simulink model "14_bus"  (R2024a)
settings: Solver=VariableStepAuto  StartTime=0.0  StopTime=1  RelTol=1e-3
undefined symbols (not defined in the file): D1, Delta
libraries: spsRMSLib x186, simulink_extras x171, spsThreePhaseVIMeasurementLib x94, spsThreePhaseBreakerLib x62, spsThreePhaseSeriesRLCBranchLib x20, spsThreePhaseSeriesRLCLoadLib x12, spsThreePhaseSourceLib x5, spsLoadFlowBusLib x5, spsStairGeneratorLib x5, spsThreePhaseTransformerTwoWindingsLib x5, spsThreePhaseFaultLib x5, sps_lib x1
(part 3 of 6)

== system 14_bus/Subsystem35 ==
  Subsystem1 : Subsystem
  Three-Phase Breaker26 : spsThreePhaseBreakerLib/Three-Phase Breaker  InitialState=closed  SwitchA=on  SwitchB=on  SwitchC=on  SwitchTimes="[1/60  5/60]"  External=on  BreakerResistance=0.01  SnubberResistance=1e6  SnubberCapacitance=inf  Measurements=None
  VI13 : spsThreePhaseVIMeasurementLib/Three-Phase V-I Measurement  VoltageMeasurement=no  SetLabelV=off  LabelV=Vabc  Vpu=off  VpuLL=off  CurrentMeasurement=yes  SetLabelI=on  LabelI=I109  Ipu=off  Pbase=100e6  Vbase=500e3  OutputType=Complex  PhasorSimulation=off  PSBequivalent=0
  A : PMIOPort  Side=Left
  B : PMIOPort  Port=2  Side=Left
  C : PMIOPort  Port=3  Side=Left
  a : PMIOPort  Port=4  Side=Right
  b : PMIOPort  Port=5  Side=Right
  c : PMIOPort  Port=6  Side=Right
  wires:
  Subsystem1/1(Out1) -> Three-Phase Breaker26/1
  [I109] -> Subsystem1/1(Iabc1)
  connections:
  VI13/LConn1 -- A/RConn1
  Three-Phase Breaker26/LConn2 -- VI13/RConn2
  Three-Phase Breaker26/LConn3 -- VI13/RConn3
  Three-Phase Breaker26/LConn1 -- VI13/RConn1
  VI13/LConn2 -- B/RConn1
  Three-Phase Breaker26/RConn1 -- a/RConn1
  VI13/LConn3 -- C/RConn1
  Three-Phase Breaker26/RConn2 -- b/RConn1
  Three-Phase Breaker26/RConn3 -- c/RConn1

== system 14_bus/Subsystem36 ==
  Subsystem1 : Subsystem
  Three-Phase Breaker26 : spsThreePhaseBreakerLib/Three-Phase Breaker  InitialState=closed  SwitchA=on  SwitchB=on  SwitchC=on  SwitchTimes="[1/60  5/60]"  External=on  BreakerResistance=0.01  SnubberResistance=1e6  SnubberCapacitance=inf  Measurements=None
  VI13 : spsThreePhaseVIMeasurementLib/Three-Phase V-I Measurement  VoltageMeasurement=no  SetLabelV=off  LabelV=Vabc  Vpu=off  VpuLL=off  CurrentMeasurement=yes  SetLabelI=on  LabelI=I910  Ipu=off  Pbase=100e6  Vbase=500e3  OutputType=Complex  PhasorSimulation=off  PSBequivalent=0
  A : PMIOPort  Side=Left
  B : PMIOPort  Port=2  Side=Left
  C : PMIOPort  Port=3  Side=Left
  a : PMIOPort  Port=4  Side=Right
  b : PMIOPort  Port=5  Side=Right
  c : PMIOPort  Port=6  Side=Right
  wires:
  Subsystem1/1(Out1) -> Three-Phase Breaker26/1
  [I910] -> Subsystem1/1(Iabc1)
  connections:
  VI13/LConn1 -- A/RConn1
  Three-Phase Breaker26/LConn2 -- VI13/RConn2
  Three-Phase Breaker26/LConn3 -- VI13/RConn3
  Three-Phase Breaker26/LConn1 -- VI13/RConn1
  VI13/LConn2 -- B/RConn1
  Three-Phase Breaker26/RConn1 -- a/RConn1
  VI13/LConn3 -- C/RConn1
  Three-Phase Breaker26/RConn2 -- b/RConn1
  Three-Phase Breaker26/RConn3 -- c/RConn1

== system 14_bus/Subsystem37 ==
  Subsystem1 : Subsystem
  Three-Phase Breaker26 : spsThreePhaseBreakerLib/Three-Phase Breaker  InitialState=closed  SwitchA=on  SwitchB=on  SwitchC=on  SwitchTimes="[1/60  5/60]"  External=on  BreakerResistance=0.01  SnubberResistance=1e6  SnubberCapacitance=inf  Measurements=None
  VI13 : spsThreePhaseVIMeasurementLib/Three-Phase V-I Measurement  VoltageMeasurement=no  SetLabelV=off  LabelV=Vabc  Vpu=off  VpuLL=off  CurrentMeasurement=yes  SetLabelI=on  LabelI=I1110  Ipu=off  Pbase=100e6  Vbase=500e3  OutputType=Complex  PhasorSimulation=off  PSBequivalent=0
  A : PMIOPort  Side=Left
  B : PMIOPort  Port=2  Side=Left
  C : PMIOPort  Port=3  Side=Left
  a : PMIOPort  Port=4  Side=Right
  b : PMIOPort  Port=5  Side=Right
  c : PMIOPort  Port=6  Side=Right
  wires:
  Subsystem1/1(Out1) -> Three-Phase Breaker26/1
  [I1110] -> Subsystem1/1(Iabc1)
  connections:
  VI13/LConn1 -- A/RConn1
  Three-Phase Breaker26/LConn2 -- VI13/RConn2
  Three-Phase Breaker26/LConn3 -- VI13/RConn3
  Three-Phase Breaker26/LConn1 -- VI13/RConn1
  VI13/LConn2 -- B/RConn1
  Three-Phase Breaker26/RConn1 -- a/RConn1
  VI13/LConn3 -- C/RConn1
  Three-Phase Breaker26/RConn2 -- b/RConn1
  Three-Phase Breaker26/RConn3 -- c/RConn1

== system 14_bus/Subsystem38 ==
  Subsystem1 : Subsystem
  Three-Phase Breaker26 : spsThreePhaseBreakerLib/Three-Phase Breaker  InitialState=closed  SwitchA=on  SwitchB=on  SwitchC=on  SwitchTimes="[1/60  5/60]"  External=on  BreakerResistance=0.01  SnubberResistance=1e6  SnubberCapacitance=inf  Measurements=None
  VI13 : spsThreePhaseVIMeasurementLib/Three-Phase V-I Measurement  VoltageMeasurement=no  SetLabelV=off  LabelV=Vabc  Vpu=off  VpuLL=off  CurrentMeasurement=yes  SetLabelI=on  LabelI=I1011  Ipu=off  Pbase=100e6  Vbase=500e3  OutputType=Complex  PhasorSimulation=off  PSBequivalent=0
  A : PMIOPort  Side=Left
  B : PMIOPort  Port=2  Side=Left
  C : PMIOPort  Port=3  Side=Left
  a : PMIOPort  Port=4  Side=Right
  b : PMIOPort  Port=5  Side=Right
  c : PMIOPort  Port=6  Side=Right
  wires:
  Subsystem1/1(Out1) -> Three-Phase Breaker26/1
  [I1011] -> Subsystem1/1(Iabc1)
  connections:
  VI13/LConn1 -- A/RConn1
  Three-Phase Breaker26/LConn2 -- VI13/RConn2
  Three-Phase Breaker26/LConn3 -- VI13/RConn3
  Three-Phase Breaker26/LConn1 -- VI13/RConn1
  VI13/LConn2 -- B/RConn1
  Three-Phase Breaker26/RConn1 -- a/RConn1
  VI13/LConn3 -- C/RConn1
  Three-Phase Breaker26/RConn2 -- b/RConn1
  Three-Phase Breaker26/RConn3 -- c/RConn1

== system 14_bus/Subsystem39 ==
  Subsystem1 : Subsystem
  Three-Phase Breaker26 : spsThreePhaseBreakerLib/Three-Phase Breaker  InitialState=closed  SwitchA=on  SwitchB=on  SwitchC=on  SwitchTimes="[1/60  5/60]"  External=on  BreakerResistance=0.01  SnubberResistance=1e6  SnubberCapacitance=inf  Measurements=None
  VI13 : spsThreePhaseVIMeasurementLib/Three-Phase V-I Measurement  VoltageMeasurement=no  SetLabelV=off  LabelV=Vabc  Vpu=off  VpuLL=off  CurrentMeasurement=yes  SetLabelI=on  LabelI=I116  Ipu=off  Pbase=100e6  Vbase=500e3  OutputType=Complex  PhasorSimulation=off  PSBequivalent=0
  A : PMIOPort  Side=Left
  B : PMIOPort  Port=2  Side=Left
  C : PMIOPort  Port=3  Side=Left
  a : PMIOPort  Port=4  Side=Right
  b : PMIOPort  Port=5  Side=Right
  c : PMIOPort  Port=6  Side=Right
  wires:
  Subsystem1/1(Out1) -> Three-Phase Breaker26/1
  [I116] -> Subsystem1/1(Iabc1)
  connections:
  VI13/LConn1 -- A/RConn1
  Three-Phase Breaker26/LConn2 -- VI13/RConn2
  Three-Phase Breaker26/LConn3 -- VI13/RConn3
  Three-Phase Breaker26/LConn1 -- VI13/RConn1
  VI13/LConn2 -- B/RConn1
  Three-Phase Breaker26/RConn1 -- a/RConn1
  VI13/LConn3 -- C/RConn1
  Three-Phase Breaker26/RConn2 -- b/RConn1
  Three-Phase Breaker26/RConn3 -- c/RConn1

== system 14_bus/Subsystem4 ==
  Subsystem25 : Subsystem
  Three-Phase Breaker26 : spsThreePhaseBreakerLib/Three-Phase Breaker  InitialState=closed  SwitchA=on  SwitchB=on  SwitchC=on  SwitchTimes="[1/60  5/60]"  External=on  BreakerResistance=0.01  SnubberResistance=1e6  SnubberCapacitance=inf  Measurements=None
  VI13 : spsThreePhaseVIMeasurementLib/Three-Phase V-I Measurement  VoltageMeasurement=no  SetLabelV=off  LabelV=Vabc  Vpu=off  VpuLL=off  CurrentMeasurement=yes  SetLabelI=on  LabelI=I74  Ipu=off  Pbase=100e6  Vbase=500e3  OutputType=Complex  PhasorSimulation=off  PSBequivalent=0
  A : PMIOPort  Side=Left
  B : PMIOPort  Port=2  Side=Left
  C : PMIOPort  Port=3  Side=Left
  a : PMIOPort  Port=4  Side=Right
  b : PMIOPort  Port=5  Side=Right
  c : PMIOPort  Port=6  Side=Right
  wires:
  Subsystem25/1(Out1) -> Three-Phase Breaker26/1
  [I74] -> Subsystem25/1(Iabc1)
  connections:
  VI13/LConn3 -- C/RConn1
  Three-Phase Breaker26/LConn3 -- VI13/RConn3
  Three-Phase Breaker26/RConn2 -- b/RConn1
  VI13/LConn1 -- A/RConn1
  Three-Phase Breaker26/RConn1 -- a/RConn1
  Three-Phase Breaker26/LConn1 -- VI13/RConn1
  Three-Phase Breaker26/LConn2 -- VI13/RConn2
  Three-Phase Breaker26/RConn3 -- c/RConn1
  VI13/LConn2 -- B/RConn1

== system 14_bus/Subsystem40 ==
  Subsystem1 : Subsystem
  Three-Phase Breaker26 : spsThreePhaseBreakerLib/Three-Phase Breaker  InitialState=closed  SwitchA=on  SwitchB=on  SwitchC=on  SwitchTimes="[1/60  5/60]"  External=on  BreakerResistance=0.01  SnubberResistance=1e6  SnubberCapacitance=inf  Measurements=None
  VI13 : spsThreePhaseVIMeasurementLib/Three-Phase V-I Measurement  VoltageMeasurement=no  SetLabelV=off  LabelV=Vabc  Vpu=off  VpuLL=off  CurrentMeasurement=yes  SetLabelI=on  LabelI=I611  Ipu=off  Pbase=100e6  Vbase=500e3  OutputType=Complex  PhasorSimulation=off  PSBequivalent=0
  A : PMIOPort  Side=Left
  B : PMIOPort  Port=2  Side=Left
  C : PMIOPort  Port=3  Side=Left
  a : PMIOPort  Port=4  Side=Right
  b : PMIOPort  Port=5  Side=Right
  c : PMIOPort  Port=6  Side=Right
  wires:
  Subsystem1/1(Out1) -> Three-Phase Breaker26/1
  [I611] -> Subsystem1/1(Iabc1)
  connections:
  VI13/LConn1 -- A/RConn1
  Three-Phase Breaker26/LConn2 -- VI13/RConn2
  Three-Phase Breaker26/LConn3 -- VI13/RConn3
  Three-Phase Breaker26/LConn1 -- VI13/RConn1
  VI13/LConn2 -- B/RConn1
  Three-Phase Breaker26/RConn1 -- a/RConn1
  VI13/LConn3 -- C/RConn1
  Three-Phase Breaker26/RConn2 -- b/RConn1
  Three-Phase Breaker26/RConn3 -- c/RConn1

== system 14_bus/Subsystem41 ==
  Subsystem1 : Subsystem
  Three-Phase Breaker26 : spsThreePhaseBreakerLib/Three-Phase Breaker  InitialState=closed  SwitchA=on  SwitchB=on  SwitchC=on  SwitchTimes="[1/60  5/60]"  External=on  BreakerResistance=0.01  SnubberResistance=1e6  SnubberCapacitance=inf  Measurements=None
  VI13 : spsThreePhaseVIMeasurementLib/Three-Phase V-I Measurement  VoltageMeasurement=no  SetLabelV=off  LabelV=Vabc  Vpu=off  VpuLL=off  CurrentMeasurement=yes  SetLabelI=on  LabelI=IL6  Ipu=off  Pbase=100e6  Vbase=500e3  OutputType=Complex  PhasorSimulation=off  PSBequivalent=0
  A : PMIOPort  Side=Left
  B : PMIOPort  Port=2  Side=Left
  C : PMIOPort  Port=3  Side=Left
  a : PMIOPort  Port=4  Side=Right
  b : PMIOPort  Port=5  Side=Right
  c : PMIOPort  Port=6  Side=Right
  wires:
  Subsystem1/1(Out1) -> Three-Phase Breaker26/1
  [IL6] -> Subsystem1/1(Iabc1)
  connections:
  VI13/LConn1 -- A/RConn1
  Three-Phase Breaker26/LConn2 -- VI13/RConn2
  Three-Phase Breaker26/LConn3 -- VI13/RConn3
  Three-Phase Breaker26/LConn1 -- VI13/RConn1
  VI13/LConn2 -- B/RConn1
  Three-Phase Breaker26/RConn1 -- a/RConn1
  VI13/LConn3 -- C/RConn1
  Three-Phase Breaker26/RConn2 -- b/RConn1
  Three-Phase Breaker26/RConn3 -- c/RConn1

== system 14_bus/Subsystem42 ==
  Subsystem1 : Subsystem
  Three-Phase Breaker26 : spsThreePhaseBreakerLib/Three-Phase Breaker  InitialState=closed  SwitchA=on  SwitchB=on  SwitchC=on  SwitchTimes="[1/60  5/60]"  External=on  BreakerResistance=0.01  SnubberResistance=1e6  SnubberCapacitance=inf  Measurements=None
  VI13 : spsThreePhaseVIMeasurementLib/Three-Phase V-I Measurement  VoltageMeasurement=no  SetLabelV=off  LabelV=Vabc  Vpu=off  VpuLL=off  CurrentMeasurement=yes  SetLabelI=on  LabelI=I56  Ipu=off  Pbase=100e6  Vbase=500e3  OutputType=Complex  PhasorSimulation=off  PSBequivalent=0
  A : PMIOPort  Side=Left
  B : PMIOPort  Port=2  Side=Left
  C : PMIOPort  Port=3  Side=Left
  a : PMIOPort  Port=4  Side=Right
  b : PMIOPort  Port=5  Side=Right
  c : PMIOPort  Port=6  Side=Right
  wires:
  Subsystem1/1(Out1) -> Three-Phase Breaker26/1
  [I56] -> Subsystem1/1(Iabc1)
  connections:
  VI13/LConn1 -- A/RConn1
  Three-Phase Breaker26/LConn2 -- VI13/RConn2
  Three-Phase Breaker26/LConn3 -- VI13/RConn3
  Three-Phase Breaker26/LConn1 -- VI13/RConn1
  VI13/LConn2 -- B/RConn1
  Three-Phase Breaker26/RConn1 -- a/RConn1
  VI13/LConn3 -- C/RConn1
  Three-Phase Breaker26/RConn2 -- b/RConn1
  Three-Phase Breaker26/RConn3 -- c/RConn1

== system 14_bus/Subsystem43 ==
  Subsystem1 : Subsystem
  Three-Phase Breaker26 : spsThreePhaseBreakerLib/Three-Phase Breaker  InitialState=closed  SwitchA=on  SwitchB=on  SwitchC=on  SwitchTimes="[1/60  5/60]"  External=on  BreakerResistance=0.01  SnubberResistance=1e6  SnubberCapacitance=inf  Measurements=None
  VI13 : spsThreePhaseVIMeasurementLib/Three-Phase V-I Measurement  VoltageMeasurement=no  SetLabelV=off  LabelV=Vabc  Vpu=off  VpuLL=off  CurrentMeasurement=yes  SetLabelI=on  LabelI=I65  Ipu=off  Pbase=100e6  Vbase=500e3  OutputType=Complex  PhasorSimulation=off  PSBequivalent=0
  A : PMIOPort  Side=Left
  B : PMIOPort  Port=2  Side=Left
  C : PMIOPort  Port=3  Side=Left
  a : PMIOPort  Port=4  Side=Right
  b : PMIOPort  Port=5  Side=Right
  c : PMIOPort  Port=6  Side=Right
  wires:
  Subsystem1/1(Out1) -> Three-Phase Breaker26/1
  [I65] -> Subsystem1/1(Iabc1)
  connections:
  VI13/LConn1 -- A/RConn1
  Three-Phase Breaker26/LConn2 -- VI13/RConn2
  Three-Phase Breaker26/LConn3 -- VI13/RConn3
  Three-Phase Breaker26/LConn1 -- VI13/RConn1
  VI13/LConn2 -- B/RConn1
  Three-Phase Breaker26/RConn1 -- a/RConn1
  VI13/LConn3 -- C/RConn1
  Three-Phase Breaker26/RConn2 -- b/RConn1
  Three-Phase Breaker26/RConn3 -- c/RConn1

== system 14_bus/Subsystem44 ==
  Subsystem1 : Subsystem
  Three-Phase Breaker26 : spsThreePhaseBreakerLib/Three-Phase Breaker  InitialState=closed  SwitchA=on  SwitchB=on  SwitchC=on  SwitchTimes="[1/60  5/60]"  External=on  BreakerResistance=0.01  SnubberResistance=1e6  SnubberCapacitance=inf  Measurements=None
  VI13 : spsThreePhaseVIMeasurementLib/Three-Phase V-I Measurement  VoltageMeasurement=no  SetLabelV=off  LabelV=Vabc  Vpu=off  VpuLL=off  CurrentMeasurement=yes  SetLabelI=on  LabelI=I149  Ipu=off  Pbase=100e6  Vbase=500e3  OutputType=Complex  PhasorSimulation=off  PSBequivalent=0
  A : PMIOPort  Side=Left
  B : PMIOPort  Port=2  Side=Left
  C : PMIOPort  Port=3  Side=Left
  a : PMIOPort  Port=4  Side=Right
  b : PMIOPort  Port=5  Side=Right
  c : PMIOPort  Port=6  Side=Right
  wires:
  Subsystem1/1(Out1) -> Three-Phase Breaker26/1
  [I149] -> Subsystem1/1(Iabc1)
  connections:
  VI13/LConn1 -- A/RConn1
  Three-Phase Breaker26/LConn2 -- VI13/RConn2
  Three-Phase Breaker26/LConn3 -- VI13/RConn3
  Three-Phase Breaker26/LConn1 -- VI13/RConn1
  VI13/LConn2 -- B/RConn1
  Three-Phase Breaker26/RConn1 -- a/RConn1
  VI13/LConn3 -- C/RConn1
  Three-Phase Breaker26/RConn2 -- b/RConn1
  Three-Phase Breaker26/RConn3 -- c/RConn1

== system 14_bus/Subsystem45 ==
  Subsystem1 : Subsystem
  Three-Phase Breaker26 : spsThreePhaseBreakerLib/Three-Phase Breaker  InitialState=closed  SwitchA=on  SwitchB=on  SwitchC=on  SwitchTimes="[1/60  5/60]"  External=on  BreakerResistance=0.01  SnubberResistance=1e6  SnubberCapacitance=inf  Measurements=None
  VI13 : spsThreePhaseVIMeasurementLib/Three-Phase V-I Measurement  VoltageMeasurement=no  SetLabelV=off  LabelV=Vabc  Vpu=off  VpuLL=off  CurrentMeasurement=yes  SetLabelI=on  LabelI=I914  Ipu=off  Pbase=100e6  Vbase=500e3  OutputType=Complex  PhasorSimulation=off  PSBequivalent=0
  A : PMIOPort  Side=Left
  B : PMIOPort  Port=2  Side=Left
  C : PMIOPort  Port=3  Side=Left
  a : PMIOPort  Port=4  Side=Right
  b : PMIOPort  Port=5  Side=Right
  c : PMIOPort  Port=6  Side=Right
  wires:
  Subsystem1/1(Out1) -> Three-Phase Breaker26/1
  [I914] -> Subsystem1/1(Iabc1)
  connections:
  VI13/LConn1 -- A/RConn1
  Three-Phase Breaker26/LConn2 -- VI13/RConn2
  Three-Phase Breaker26/LConn3 -- VI13/RConn3
  Three-Phase Breaker26/LConn1 -- VI13/RConn1
  VI13/LConn2 -- B/RConn1
  Three-Phase Breaker26/RConn1 -- a/RConn1
  VI13/LConn3 -- C/RConn1
  Three-Phase Breaker26/RConn2 -- b/RConn1
  Three-Phase Breaker26/RConn3 -- c/RConn1

== system 14_bus/Subsystem46 ==
  Subsystem1 : Subsystem
  Three-Phase Breaker26 : spsThreePhaseBreakerLib/Three-Phase Breaker  InitialState=closed  SwitchA=on  SwitchB=on  SwitchC=on  SwitchTimes="[1/60  5/60]"  External=on  BreakerResistance=0.01  SnubberResistance=1e6  SnubberCapacitance=inf  Measurements=None
  VI13 : spsThreePhaseVIMeasurementLib/Three-Phase V-I Measurement  VoltageMeasurement=no  SetLabelV=off  LabelV=Vabc  Vpu=off  VpuLL=off  CurrentMeasurement=yes  SetLabelI=on  LabelI=I1413  Ipu=off  Pbase=100e6  Vbase=500e3  OutputType=Complex  PhasorSimulation=off  PSBequivalent=0
  A : PMIOPort  Side=Left
  B : PMIOPort  Port=2  Side=Left
  C : PMIOPort  Port=3  Side=Left
  a : PMIOPort  Port=4  Side=Right
  b : PMIOPort  Port=5  Side=Right
  c : PMIOPort  Port=6  Side=Right
  wires:
  Subsystem1/1(Out1) -> Three-Phase Breaker26/1
  [I1413] -> Subsystem1/1(Iabc1)
  connections:
  VI13/LConn1 -- A/RConn1
  Three-Phase Breaker26/LConn2 -- VI13/RConn2
  Three-Phase Breaker26/LConn3 -- VI13/RConn3
  Three-Phase Breaker26/LConn1 -- VI13/RConn1
  VI13/LConn2 -- B/RConn1
  Three-Phase Breaker26/RConn1 -- a/RConn1
  VI13/LConn3 -- C/RConn1
  Three-Phase Breaker26/RConn2 -- b/RConn1
  Three-Phase Breaker26/RConn3 -- c/RConn1

== system 14_bus/Subsystem47 ==
  Subsystem1 : Subsystem
  Three-Phase Breaker26 : spsThreePhaseBreakerLib/Three-Phase Breaker  InitialState=closed  SwitchA=on  SwitchB=on  SwitchC=on  SwitchTimes="[1/60  5/60]"  External=on  BreakerResistance=0.01  SnubberResistance=1e6  SnubberCapacitance=inf  Measurements=None
  VI13 : spsThreePhaseVIMeasurementLib/Three-Phase V-I Measurement  VoltageMeasurement=no  SetLabelV=off  LabelV=Vabc  Vpu=off  VpuLL=off  CurrentMeasurement=yes  SetLabelI=on  LabelI=I1314  Ipu=off  Pbase=100e6  Vbase=500e3  OutputType=Complex  PhasorSimulation=off  PSBequivalent=0
  A : PMIOPort  Side=Left
  B : PMIOPort  Port=2  Side=Left
  C : PMIOPort  Port=3  Side=Left
  a : PMIOPort  Port=4  Side=Right
  b : PMIOPort  Port=5  Side=Right
  c : PMIOPort  Port=6  Side=Right
  wires:
  Subsystem1/1(Out1) -> Three-Phase Breaker26/1
  [I1314] -> Subsystem1/1(Iabc1)
  connections:
  VI13/LConn1 -- A/RConn1
  Three-Phase Breaker26/LConn2 -- VI13/RConn2
  Three-Phase Breaker26/LConn3 -- VI13/RConn3
  Three-Phase Breaker26/LConn1 -- VI13/RConn1
  VI13/LConn2 -- B/RConn1
  Three-Phase Breaker26/RConn1 -- a/RConn1
  VI13/LConn3 -- C/RConn1
  Three-Phase Breaker26/RConn2 -- b/RConn1
  Three-Phase Breaker26/RConn3 -- c/RConn1

== system 14_bus/Subsystem48 ==
  Subsystem1 : Subsystem
  Three-Phase Breaker26 : spsThreePhaseBreakerLib/Three-Phase Breaker  InitialState=closed  SwitchA=on  SwitchB=on  SwitchC=on  SwitchTimes="[1/60  5/60]"  External=on  BreakerResistance=0.01  SnubberResistance=1e6  SnubberCapacitance=inf  Measurements=None
  VI13 : spsThreePhaseVIMeasurementLib/Three-Phase V-I Measurement  VoltageMeasurement=no  SetLabelV=off  LabelV=Vabc  Vpu=off  VpuLL=off  CurrentMeasurement=yes  SetLabelI=on  LabelI=IL14  Ipu=off  Pbase=100e6  Vbase=500e3  OutputType=Complex  PhasorSimulation=off  PSBequivalent=0
  A : PMIOPort  Side=Left
  B : PMIOPort  Port=2  Side=Left
  C : PMIOPort  Port=3  Side=Left
  a : PMIOPort  Port=4  Side=Right
  b : PMIOPort  Port=5  Side=Right
  c : PMIOPort  Port=6  Side=Right
  wires:
  Subsystem1/1(Out1) -> Three-Phase Breaker26/1
  [IL14] -> Subsystem1/1(Iabc1)
  connections:
  VI13/LConn1 -- A/RConn1
  Three-Phase Breaker26/LConn2 -- VI13/RConn2
  Three-Phase Breaker26/LConn3 -- VI13/RConn3
  Three-Phase Breaker26/LConn1 -- VI13/RConn1
  VI13/LConn2 -- B/RConn1
  Three-Phase Breaker26/RConn1 -- a/RConn1
  VI13/LConn3 -- C/RConn1
  Three-Phase Breaker26/RConn2 -- b/RConn1
  Three-Phase Breaker26/RConn3 -- c/RConn1

== system 14_bus/Subsystem49 ==
  Subsystem1 : Subsystem
  Three-Phase Breaker26 : spsThreePhaseBreakerLib/Three-Phase Breaker  InitialState=closed  SwitchA=on  SwitchB=on  SwitchC=on  SwitchTimes="[1/60  5/60]"  External=on  BreakerResistance=0.01  SnubberResistance=1e6  SnubberCapacitance=inf  Measurements=None
  VI13 : spsThreePhaseVIMeasurementLib/Three-Phase V-I Measurement  VoltageMeasurement=no  SetLabelV=off  LabelV=Vabc  Vpu=off  VpuLL=off  CurrentMeasurement=yes  SetLabelI=on  LabelI=IL13  Ipu=off  Pbase=100e6  Vbase=500e3  OutputType=Complex  PhasorSimulation=off  PSBequivalent=0
  A : PMIOPort  Side=Left
  B : PMIOPort  Port=2  Side=Left
  C : PMIOPort  Port=3  Side=Left
  a : PMIOPort  Port=4  Side=Right
  b : PMIOPort  Port=5  Side=Right
  c : PMIOPort  Port=6  Side=Right
  wires:
  Subsystem1/1(Out1) -> Three-Phase Breaker26/1
  [IL13] -> Subsystem1/1(Iabc1)
  connections:
  VI13/LConn1 -- A/RConn1
  Three-Phase Breaker26/LConn2 -- VI13/RConn2
  Three-Phase Breaker26/LConn3 -- VI13/RConn3
  Three-Phase Breaker26/LConn1 -- VI13/RConn1
  VI13/LConn2 -- B/RConn1
  Three-Phase Breaker26/RConn1 -- a/RConn1
  VI13/LConn3 -- C/RConn1
  Three-Phase Breaker26/RConn2 -- b/RConn1
  Three-Phase Breaker26/RConn3 -- c/RConn1

== system 14_bus/Subsystem5 ==
  Subsystem1 : Subsystem
  Three-Phase Breaker26 : spsThreePhaseBreakerLib/Three-Phase Breaker  InitialState=closed  SwitchA=on  SwitchB=on  SwitchC=on  SwitchTimes="[1/60  5/60]"  External=on  BreakerResistance=0.01  SnubberResistance=1e6  SnubberCapacitance=inf  Measurements=None
  VI13 : spsThreePhaseVIMeasurementLib/Three-Phase V-I Measurement  VoltageMeasurement=no  SetLabelV=off  LabelV=Vabc  Vpu=off  VpuLL=off  CurrentMeasurement=yes  SetLabelI=on  LabelI=I21  Ipu=off  Pbase=100e6  Vbase=500e3  OutputType=Complex  PhasorSimulation=off  PSBequivalent=0
  A : PMIOPort  Side=Left
  B : PMIOPort  Port=2  Side=Left
  C : PMIOPort  Port=3  Side=Left
  a : PMIOPort  Port=4  Side=Right
  b : PMIOPort  Port=5  Side=Right
  c : PMIOPort  Port=6  Side=Right
  wires:
  Subsystem1/1(Out1) -> Three-Phase Breaker26/1
  [I21] -> Subsystem1/1(Iabc1)
  connections:
  VI13/LConn1 -- A/RConn1
  Three-Phase Breaker26/LConn2 -- VI13/RConn2
  Three-Phase Breaker26/LConn3 -- VI13/RConn3
  Three-Phase Breaker26/LConn1 -- VI13/RConn1
  VI13/LConn2 -- B/RConn1
  Three-Phase Breaker26/RConn1 -- a/RConn1
  VI13/LConn3 -- C/RConn1
  Three-Phase Breaker26/RConn2 -- b/RConn1
  Three-Phase Breaker26/RConn3 -- c/RConn1

== system 14_bus/Subsystem50 ==
  Subsystem1 : Subsystem
  Three-Phase Breaker26 : spsThreePhaseBreakerLib/Three-Phase Breaker  InitialState=closed  SwitchA=on  SwitchB=on  SwitchC=on  SwitchTimes="[1/60  5/60]"  External=on  BreakerResistance=0.01  SnubberResistance=1e6  SnubberCapacitance=inf  Measurements=None
  VI13 : spsThreePhaseVIMeasurementLib/Three-Phase V-I Measurement  VoltageMeasurement=no  SetLabelV=off  LabelV=Vabc  Vpu=off  VpuLL=off  CurrentMeasurement=yes  SetLabelI=on  LabelI=IL12  Ipu=off  Pbase=100e6  Vbase=500e3  OutputType=Complex  PhasorSimulation=off  PSBequivalent=0
  A : PMIOPort  Side=Left
  B : PMIOPort  Port=2  Side=Left
  C : PMIOPort  Port=3  Side=Left
  a : PMIOPort  Port=4  Side=Right
  b : PMIOPort  Port=5  Side=Right
  c : PMIOPort  Port=6  Side=Right
  wires:
  Subsystem1/1(Out1) -> Three-Phase Breaker26/1
  [IL12] -> Subsystem1/1(Iabc1)
  connections:
  VI13/LConn1 -- A/RConn1
  Three-Phase Breaker26/LConn2 -- VI13/RConn2
  Three-Phase Breaker26/LConn3 -- VI13/RConn3
  Three-Phase Breaker26/LConn1 -- VI13/RConn1
  VI13/LConn2 -- B/RConn1
  Three-Phase Breaker26/RConn1 -- a/RConn1
  VI13/LConn3 -- C/RConn1
  Three-Phase Breaker26/RConn2 -- b/RConn1
  Three-Phase Breaker26/RConn3 -- c/RConn1

== system 14_bus/Subsystem51 ==
  Subsystem1 : Subsystem
  Three-Phase Breaker26 : spsThreePhaseBreakerLib/Three-Phase Breaker  InitialState=closed  SwitchA=on  SwitchB=on  SwitchC=on  SwitchTimes="[1/60  5/60]"  External=on  BreakerResistance=0.01  SnubberResistance=1e6  SnubberCapacitance=inf  Measurements=None
  VI13 : spsThreePhaseVIMeasurementLib/Three-Phase V-I Measurement  VoltageMeasurement=no  SetLabelV=off  LabelV=Vabc  Vpu=off  VpuLL=off  CurrentMeasurement=yes  SetLabelI=on  LabelI=I1312  Ipu=off  Pbase=100e6  Vbase=500e3  OutputType=Complex  PhasorSimulation=off  PSBequivalent=0
  A : PMIOPort  Side=Left
  B : PMIOPort  Port=2  Side=Left
  C : PMIOPort  Port=3  Side=Left
  a : PMIOPort  Port=4  Side=Right
  b : PMIOPort  Port=5  Side=Right
  c : PMIOPort  Port=6  Side=Right
  wires:
  Subsystem1/1(Out1) -> Three-Phase Breaker26/1
  [I1312] -> Subsystem1/1(Iabc1)
  connections:
  VI13/LConn1 -- A/RConn1
  Three-Phase Breaker26/LConn2 -- VI13/RConn2
  Three-Phase Breaker26/LConn3 -- VI13/RConn3
  Three-Phase Breaker26/LConn1 -- VI13/RConn1
  VI13/LConn2 -- B/RConn1
  Three-Phase Breaker26/RConn1 -- a/RConn1
  VI13/LConn3 -- C/RConn1
  Three-Phase Breaker26/RConn2 -- b/RConn1
  Three-Phase Breaker26/RConn3 -- c/RConn1

== system 14_bus/Subsystem52 ==
  Subsystem1 : Subsystem
  Three-Phase Breaker26 : spsThreePhaseBreakerLib/Three-Phase Breaker  InitialState=closed  SwitchA=on  SwitchB=on  SwitchC=on  SwitchTimes="[1/60  5/60]"  External=on  BreakerResistance=0.01  SnubberResistance=1e6  SnubberCapacitance=inf  Measurements=None
  VI13 : spsThreePhaseVIMeasurementLib/Three-Phase V-I Measurement  VoltageMeasurement=no  SetLabelV=off  LabelV=Vabc  Vpu=off  VpuLL=off  CurrentMeasurement=yes  SetLabelI=on  LabelI=I1213  Ipu=off  Pbase=100e6  Vbase=500e3  OutputType=Complex  PhasorSimulation=off  PSBequivalent=0
  A : PMIOPort  Side=Left
  B : PMIOPort  Port=2  Side=Left
  C : PMIOPort  Port=3  Side=Left
  a : PMIOPort  Port=4  Side=Right
  b : PMIOPort  Port=5  Side=Right
  c : PMIOPort  Port=6  Side=Right
  wires:
  Subsystem1/1(Out1) -> Three-Phase Breaker26/1
  [I1213] -> Subsystem1/1(Iabc1)
  connections:
  VI13/LConn1 -- A/RConn1
  Three-Phase Breaker26/LConn2 -- VI13/RConn2
  Three-Phase Breaker26/LConn3 -- VI13/RConn3
  Three-Phase Breaker26/LConn1 -- VI13/RConn1
  VI13/LConn2 -- B/RConn1
  Three-Phase Breaker26/RConn1 -- a/RConn1
  VI13/LConn3 -- C/RConn1
  Three-Phase Breaker26/RConn2 -- b/RConn1
  Three-Phase Breaker26/RConn3 -- c/RConn1

== system 14_bus/Subsystem53 ==
  Subsystem1 : Subsystem
  Three-Phase Breaker26 : spsThreePhaseBreakerLib/Three-Phase Breaker  InitialState=closed  SwitchA=on  SwitchB=on  SwitchC=on  SwitchTimes="[1/60  5/60]"  External=on  BreakerResistance=0.01  SnubberResistance=1e6  SnubberCapacitance=inf  Measurements=None
  VI13 : spsThreePhaseVIMeasurementLib/Three-Phase V-I Measurement  VoltageMeasurement=no  SetLabelV=off  LabelV=Vabc  Vpu=off  VpuLL=off  CurrentMeasurement=yes  SetLabelI=on  LabelI=I126  Ipu=off  Pbase=100e6  Vbase=500e3  OutputType=Complex  PhasorSimulation=off  PSBequivalent=0
  A : PMIOPort  Side=Left
  B : PMIOPort  Port=2  Side=Left
  C : PMIOPort  Port=3  Side=Left
  a : PMIOPort  Port=4  Side=Right
  b : PMIOPort  Port=5  Side=Right
  c : PMIOPort  Port=6  Side=Right
  wires:
  Subsystem1/1(Out1) -> Three-Phase Breaker26/1
  [I126] -> Subsystem1/1(Iabc1)
  connections:
  VI13/LConn1 -- A/RConn1
  Three-Phase Breaker26/LConn2 -- VI13/RConn2
  Three-Phase Breaker26/LConn3 -- VI13/RConn3
  Three-Phase Breaker26/LConn1 -- VI13/RConn1
  VI13/LConn2 -- B/RConn1
  Three-Phase Breaker26/RConn1 -- a/RConn1
  VI13/LConn3 -- C/RConn1
  Three-Phase Breaker26/RConn2 -- b/RConn1
  Three-Phase Breaker26/RConn3 -- c/RConn1

== system 14_bus/Subsystem54 ==
  Subsystem1 : Subsystem
  Three-Phase Breaker26 : spsThreePhaseBreakerLib/Three-Phase Breaker  InitialState=closed  SwitchA=on  SwitchB=on  SwitchC=on  SwitchTimes="[1/60  5/60]"  External=on  BreakerResistance=0.01  SnubberResistance=1e6  SnubberCapacitance=inf  Measurements=None
  VI13 : spsThreePhaseVIMeasurementLib/Three-Phase V-I Measurement  VoltageMeasurement=no  SetLabelV=off  LabelV=Vabc  Vpu=off  VpuLL=off  CurrentMeasurement=yes  SetLabelI=on  LabelI=I612  Ipu=off  Pbase=100e6  Vbase=500e3  OutputType=Complex  PhasorSimulation=off  PSBequivalent=0
  A : PMIOPort  Side=Left
  B : PMIOPort  Port=2  Side=Left
  C : PMIOPort  Port=3  Side=Left
  a : PMIOPort  Port=4  Side=Right
  b : PMIOPort  Port=5  Side=Right
  c : PMIOPort  Port=6  Side=Right
  wires:
  Subsystem1/1(Out1) -> Three-Phase Breaker26/1
  [I612] -> Subsystem1/1(Iabc1)
  connections:
  VI13/LConn1 -- A/RConn1
  Three-Phase Breaker26/LConn2 -- VI13/RConn2
  Three-Phase Breaker26/LConn3 -- VI13/RConn3
  Three-Phase Breaker26/LConn1 -- VI13/RConn1
  VI13/LConn2 -- B/RConn1
  Three-Phase Breaker26/RConn1 -- a/RConn1
  VI13/LConn3 -- C/RConn1
  Three-Phase Breaker26/RConn2 -- b/RConn1
  Three-Phase Breaker26/RConn3 -- c/RConn1

== system 14_bus/Subsystem55 ==
  Subsystem1 : Subsystem
  Three-Phase Breaker26 : spsThreePhaseBreakerLib/Three-Phase Breaker  InitialState=closed  SwitchA=on  SwitchB=on  SwitchC=on  SwitchTimes="[1/60  5/60]"  External=on  BreakerResistance=0.01  SnubberResistance=1e6  SnubberCapacitance=inf  Measurements=None
  VI13 : spsThreePhaseVIMeasurementLib/Three-Phase V-I Measurement  VoltageMeasurement=no  SetLabelV=off  LabelV=Vabc  Vpu=off  VpuLL=off  CurrentMeasurement=yes  SetLabelI=on  LabelI=I136  Ipu=off  Pbase=100e6  Vbase=500e3  OutputType=Complex  PhasorSimulation=off  PSBequivalent=0
  A : PMIOPort  Side=Left
  B : PMIOPort  Port=2  Side=Left
  C : PMIOPort  Port=3  Side=Left
  a : PMIOPort  Port=4  Side=Right
  b : PMIOPort  Port=5  Side=Right
  c : PMIOPort  Port=6  Side=Right
  wires:
  Subsystem1/1(Out1) -> Three-Phase Breaker26/1
  [I136] -> Subsystem1/1(Iabc1)
  connections:
  VI13/LConn1 -- A/RConn1
  Three-Phase Breaker26/LConn2 -- VI13/RConn2
  Three-Phase Breaker26/LConn3 -- VI13/RConn3
  Three-Phase Breaker26/LConn1 -- VI13/RConn1
  VI13/LConn2 -- B/RConn1
  Three-Phase Breaker26/RConn1 -- a/RConn1
  VI13/LConn3 -- C/RConn1
  Three-Phase Breaker26/RConn2 -- b/RConn1
  Three-Phase Breaker26/RConn3 -- c/RConn1

== system 14_bus/Subsystem56 ==
  Subsystem1 : Subsystem
  Three-Phase Breaker26 : spsThreePhaseBreakerLib/Three-Phase Breaker  InitialState=closed  SwitchA=on  SwitchB=on  SwitchC=on  SwitchTimes="[1/60  5/60]"  External=on  BreakerResistance=0.01  SnubberResistance=1e6  SnubberCapacitance=inf  Measurements=None
  VI13 : spsThreePhaseVIMeasurementLib/Three-Phase V-I Measurement  VoltageMeasurement=no  SetLabelV=off  LabelV=Vabc  Vpu=off  VpuLL=off  CurrentMeasurement=yes  SetLabelI=on  LabelI=I613  Ipu=off  Pbase=100e6  Vbase=500e3  OutputType=Complex  PhasorSimulation=off  PSBequivalent=0
  A : PMIOPort  Side=Left
  B : PMIOPort  Port=2  Side=Left
  C : PMIOPort  Port=3  Side=Left
  a : PMIOPort  Port=4  Side=Right
  b : PMIOPort  Port=5  Side=Right
  c : PMIOPort  Port=6  Side=Right
  wires:
  Subsystem1/1(Out1) -> Three-Phase Breaker26/1
  [I613] -> Subsystem1/1(Iabc1)
  connections:
  VI13/LConn1 -- A/RConn1
  Three-Phase Breaker26/LConn2 -- VI13/RConn2
  Three-Phase Breaker26/LConn3 -- VI13/RConn3
  Three-Phase Breaker26/LConn1 -- VI13/RConn1
  VI13/LConn2 -- B/RConn1
  Three-Phase Breaker26/RConn1 -- a/RConn1
  VI13/LConn3 -- C/RConn1
  Three-Phase Breaker26/RConn2 -- b/RConn1
  Three-Phase Breaker26/RConn3 -- c/RConn1

== system 14_bus/Subsystem57 ==
  Subsystem1 : Subsystem
  Three-Phase Breaker26 : spsThreePhaseBreakerLib/Three-Phase Breaker  InitialState=closed  SwitchA=on  SwitchB=on  SwitchC=on  SwitchTimes="[1/60  5/60]"  External=on  BreakerResistance=0.01  SnubberResistance=1e6  SnubberCapacitance=inf  Measurements=None
  VI13 : spsThreePhaseVIMeasurementLib/Three-Phase V-I Measurement  VoltageMeasurement=no  SetLabelV=off  LabelV=Vabc  Vpu=off  VpuLL=off  CurrentMeasurement=yes  SetLabelI=on  LabelI=IL10  Ipu=off  Pbase=100e6  Vbase=500e3  OutputType=Complex  PhasorSimulation=off  PSBequivalent=0
  A : PMIOPort  Side=Left
  B : PMIOPort  Port=2  Side=Left
  C : PMIOPort  Port=3  Side=Left
  a : PMIOPort  Port=4  Side=Right
  b : PMIOPort  Port=5  Side=Right
  c : PMIOPort  Port=6  Side=Right
  wires:
  Subsystem1/1(Out1) -> Three-Phase Breaker26/1
  [IL10] -> Subsystem1/1(Iabc1)
  connections:
  VI13/LConn1 -- A/RConn1
  Three-Phase Breaker26/LConn2 -- VI13/RConn2
  Three-Phase Breaker26/LConn3 -- VI13/RConn3
  Three-Phase Breaker26/LConn1 -- VI13/RConn1
  VI13/LConn2 -- B/RConn1
  Three-Phase Breaker26/RConn1 -- a/RConn1
  VI13/LConn3 -- C/RConn1
  Three-Phase Breaker26/RConn2 -- b/RConn1
  Three-Phase Breaker26/RConn3 -- c/RConn1

== system 14_bus/Subsystem58 ==
  Subsystem1 : Subsystem
  Three-Phase Breaker26 : spsThreePhaseBreakerLib/Three-Phase Breaker  InitialState=closed  SwitchA=on  SwitchB=on  SwitchC=on  SwitchTimes="[1/60  5/60]"  External=on  BreakerResistance=0.01  SnubberResistance=1e6  SnubberCapacitance=inf  Measurements=None
  VI13 : spsThreePhaseVIMeasurementLib/Three-Phase V-I Measurement  VoltageMeasurement=no  SetLabelV=off  LabelV=Vabc  Vpu=off  VpuLL=off  CurrentMeasurement=yes  SetLabelI=on  LabelI=IL11  Ipu=off  Pbase=100e6  Vbase=500e3  OutputType=Complex  PhasorSimulation=off  PSBequivalent=0
  A : PMIOPort  Side=Left
  B : PMIOPort  Port=2  Side=Left
  C : PMIOPort  Port=3  Side=Left
  a : PMIOPort  Port=4  Side=Right
  b : PMIOPort  Port=5  Side=Right
  c : PMIOPort  Port=6  Side=Right
  wires:
  Subsystem1/1(Out1) -> Three-Phase Breaker26/1
  [IL11] -> Subsystem1/1(Iabc1)
  connections:
  VI13/LConn1 -- A/RConn1
  Three-Phase Breaker26/LConn2 -- VI13/RConn2
  Three-Phase Breaker26/LConn3 -- VI13/RConn3
  Three-Phase Breaker26/LConn1 -- VI13/RConn1
  VI13/LConn2 -- B/RConn1
  Three-Phase Breaker26/RConn1 -- a/RConn1
  VI13/LConn3 -- C/RConn1
  Three-Phase Breaker26/RConn2 -- b/RConn1
  Three-Phase Breaker26/RConn3 -- c/RConn1

== system 14_bus/Subsystem6 ==
  Subsystem1 : Subsystem
  Three-Phase Breaker26 : spsThreePhaseBreakerLib/Three-Phase Breaker  InitialState=closed  SwitchA=on  SwitchB=on  SwitchC=on  SwitchTimes="[1/60  5/60]"  External=on  BreakerResistance=0.01  SnubberResistance=1e6  SnubberCapacitance=inf  Measurements=None
  VI13 : spsThreePhaseVIMeasurementLib/Three-Phase V-I Measurement  VoltageMeasurement=no  SetLabelV=off  LabelV=Vabc  Vpu=off  VpuLL=off  CurrentMeasurement=yes  SetLabelI=on  LabelI=I12  Ipu=off  Pbase=100e6  Vbase=500e3  OutputType=Complex  PhasorSimulation=off  PSBequivalent=0
  A : PMIOPort  Side=Left
  B : PMIOPort  Port=2  Side=Left
  C : PMIOPort  Port=3  Side=Left
  a : PMIOPort  Port=4  Side=Right
  b : PMIOPort  Port=5  Side=Right
  c : PMIOPort  Port=6  Side=Right
  wires:
  Subsystem1/1(Out1) -> Three-Phase Breaker26/1
  [I12] -> Subsystem1/1(Iabc1)
  connections:
  VI13/LConn1 -- A/RConn1
  Three-Phase Breaker26/LConn2 -- VI13/RConn2
  Three-Phase Breaker26/LConn3 -- VI13/RConn3
  Three-Phase Breaker26/LConn1 -- VI13/RConn1
  VI13/LConn2 -- B/RConn1
  Three-Phase Breaker26/RConn1 -- a/RConn1
  VI13/LConn3 -- C/RConn1
  Three-Phase Breaker26/RConn2 -- b/RConn1
  Three-Phase Breaker26/RConn3 -- c/RConn1

== system 14_bus/Subsystem7 ==
  Subsystem11 : Subsystem
  Three-Phase Breaker11 : spsThreePhaseBreakerLib/Three-Phase Breaker  InitialState=closed  SwitchA=on  SwitchB=on  SwitchC=on  SwitchTimes="[1/60  5/60]"  External=on  BreakerResistance=0.01  SnubberResistance=1e6  SnubberCapacitance=inf  Measurements=None
  VI3 : spsThreePhaseVIMeasurementLib/Three-Phase V-I Measurement  VoltageMeasurement=no  SetLabelV=off  LabelV=Vabc  Vpu=off  VpuLL=off  CurrentMeasurement=yes  SetLabelI=on  LabelI=IL3  Ipu=off  Pbase=100e6  Vbase=500e3  OutputType=Complex  PhasorSimulation=off  PSBequivalent=0
  c : PMIOPort  Side=Right
  b : PMIOPort  Port=2  Side=Right
  a : PMIOPort  Port=3  Side=Right
  C : PMIOPort  Port=4  Side=Left
  B : PMIOPort  Port=5  Side=Left
  A : PMIOPort  Port=6  Side=Left
  wires:
  Subsystem11/1(Out1) -> Three-Phase Breaker11/1
  [IL3] -> Subsystem11/1(Iabc1)
  connections:
  C/RConn1 -- VI3/LConn3
  Three-Phase Breaker11/RConn2 -- b/RConn1
  VI3/RConn2 -- Three-Phase Breaker11/LConn2
  Three-Phase Breaker11/RConn3 -- c/RConn1
  VI3/RConn3 -- Three-Phase Breaker11/LConn3
  A/RConn1 -- VI3/LConn1
  Three-Phase Breaker11/RConn1 -- a/RConn1
  VI3/LConn2 -- B/RConn1
  Three-Phase Breaker11/LConn1 -- VI3/RConn1

== system 14_bus/Subsystem8 ==
  Vabc : Inport
  Vabc1 : Inport  Port=2
  Subsystem7 : Subsystem
  Three-Phase Transformer (Two Windings)1 : spsThreePhaseTransformerTwoWindingsLib/Three-Phase Transformer (Two Windings)  Winding1Connection=Delta (D1)  Winding2Connection=Yg  CoreType=Three single-phase transformers  SetSaturation=off  Hysteresis=off  DataFile='hysteresis'  SetInitialFlux=off  Measurements=None  UNITS=pu  NominalPower=[ 250e6 , 50 ]  Winding1=[25e3*1.045 , 0.002 , 0.08 ]  Winding2=[ 25e3*1.045 , 0.002 , 0.08 ]  Rm=500  Lm=500  L0=0.5  Saturation=[ 0,0 ; 0.0024,1.2 ; 1.0,1.52 ]  InitialFluxes=[ 0.8 , -0.8 , 0.7 ]  BreakLoop=off  DiscreteSolver=Trapezoidal iterative  DataType=off  TransfoNumber=1
  Three-Phase Breaker6 : spsThreePhaseBreakerLib/Three-Phase Breaker  InitialState=closed  SwitchA=on  SwitchB=on  SwitchC=on  SwitchTimes="[1/60  5/60]"  External=on  BreakerResistance=0.01  SnubberResistance=1e6  SnubberCapacitance=inf  Measurements=None
  Three-Phase Breaker7 : spsThreePhaseBreakerLib/Three-Phase Breaker  InitialState=closed  SwitchA=on  SwitchB=on  SwitchC=on  SwitchTimes="[1/60  5/60]"  External=on  BreakerResistance=0.01  SnubberResistance=1e6  SnubberCapacitance=inf  Measurements=None
  a : PMIOPort  Side=Right
  b : PMIOPort  Port=2  Side=Right
  c : PMIOPort  Port=3  Side=Right
  C : PMIOPort  Port=4  Side=Left
  B : PMIOPort  Port=5  Side=Left
  A : PMIOPort  Port=6  Side=Left
  wires:
  Subsystem7/1(Out1) -> Three-Phase Breaker7/1, Three-Phase Breaker6/1
  Vabc/1 -> Subsystem7/2(Vabc)
  Vabc1/1 -> Subsystem7/1(Vabc1)
  connections:
  Three-Phase Transformer (Two Windings)1/LConn2 -- Three-Phase Breaker7/RConn2
  Three-Phase Breaker7/RConn1 -- Three-Phase Transformer (Two Windings)1/LConn1
  Three-Phase Transformer (Two Windings)1/RConn2 -- Three-Phase Breaker6/LConn2
  Three-Phase Breaker6/RConn3 -- c/RConn1
  Three-Phase Breaker6/LConn1 -- Three-Phase Transformer (Two Windings)1/RConn1
  Three-Phase Breaker7/RConn3 -- Three-Phase Transformer (Two Windings)1/LConn3
  Three-Phase Transformer (Two Windings)1/RConn3 -- Three-Phase Breaker6/LConn3
  C/RConn1 -- Three-Phase Breaker7/LConn3
  B/RConn1 -- Three-Phase Breaker7/LConn2
  Three-Phase Breaker7/LConn1 -- A/RConn1
  Three-Phase Breaker6/RConn2 -- b/RConn1
  Three-Phase Breaker6/RConn1 -- a/RConn1

== system 14_bus/Subsystem9 ==
  Subsystem1 : Subsystem
  Three-Phase Breaker26 : spsThreePhaseBreakerLib/Three-Phase Breaker  InitialState=closed  SwitchA=on  SwitchB=on  SwitchC=on  SwitchTimes="[1/60  5/60]"  External=on  BreakerResistance=0.01  SnubberResistance=1e6  SnubberCapacitance=inf  Measurements=None
  VI13 : spsThreePhaseVIMeasurementLib/Three-Phase V-I Measurement  VoltageMeasurement=no  SetLabelV=off  LabelV=Vabc  Vpu=off  VpuLL=off  CurrentMeasurement=yes  SetLabelI=on  LabelI=I32  Ipu=off  Pbase=100e6  Vbase=500e3  OutputType=Complex  PhasorSimulation=off  PSBequivalent=0
  A : PMIOPort  Side=Left
  B : PMIOPort  Port=2  Side=Left
  C : PMIOPort  Port=3  Side=Left
  a : PMIOPort  Port=4  Side=Right
  b : PMIOPort  Port=5  Side=Right
  c : PMIOPort  Port=6  Side=Right
  wires:
  Subsystem1/1(Out1) -> Three-Phase Breaker26/1
  [I32] -> Subsystem1/1(Iabc1)
  connections:
  VI13/LConn1 -- A/RConn1
  Three-Phase Breaker26/LConn2 -- VI13/RConn2
  Three-Phase Breaker26/LConn3 -- VI13/RConn3
  Three-Phase Breaker26/LConn1 -- VI13/RConn1
  VI13/LConn2 -- B/RConn1
  Three-Phase Breaker26/RConn1 -- a/RConn1
  VI13/LConn3 -- C/RConn1
  Three-Phase Breaker26/RConn2 -- b/RConn1
  Three-Phase Breaker26/RConn3 -- c/RConn1

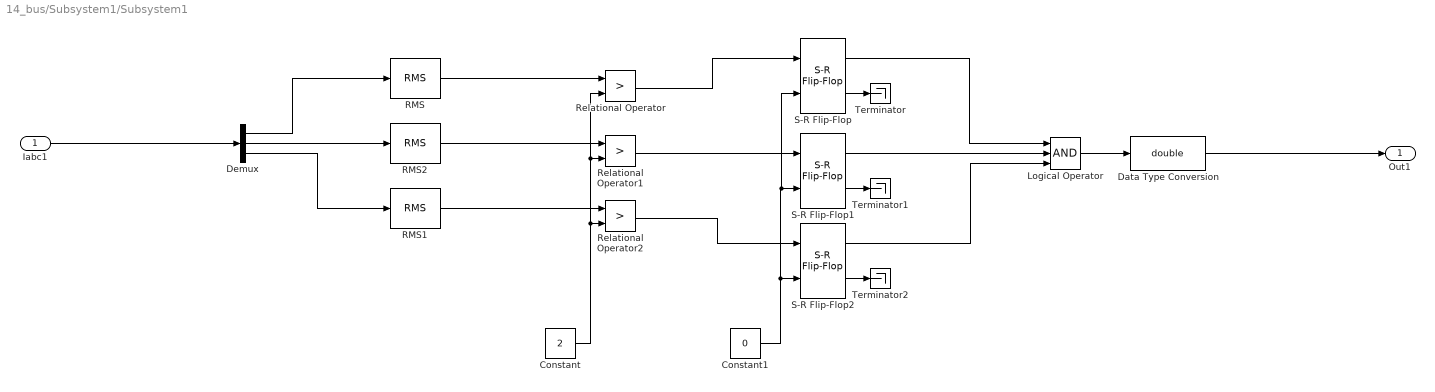
== system 14_bus/Subsystem1/Subsystem1 ==
  Iabc1 : Inport
  Constant : Constant  Value=2  OutDataTypeStr=boolean
  Constant1 : Constant  Value=0  OutDataTypeStr=boolean
  Data Type Conversion : DataTypeConversion  OutDataTypeStr=double  SaturateOnIntegerOverflow=off  RndMeth=Floor
  Demux : Demux  Outputs=3
  Logical Operator : Logic  Inputs=3  AllPortsSameDT=off  OutDataTypeStr=boolean
  RMS : spsRMSLib/RMS  TrueRMS=on  Freq=60  RMSInit=120  Ts=0
  RMS1 : spsRMSLib/RMS  TrueRMS=on  Freq=60  RMSInit=120  Ts=0
  RMS2 : spsRMSLib/RMS  TrueRMS=on  Freq=60  RMSInit=120  Ts=0
  Relational Operator : RelationalOperator  Operator=>  OutDataTypeStr=boolean  RndMeth=Simplest  InputSameDT=off
  Relational Operator1 : RelationalOperator  Operator=>  OutDataTypeStr=boolean  RndMeth=Simplest  InputSameDT=off
  Relational Operator2 : RelationalOperator  Operator=>  OutDataTypeStr=boolean  RndMeth=Simplest  InputSameDT=off
  S-R Flip-Flop : simulink_extras/Flip Flops/S-R Flip-Flop  initial_condition=0
  S-R Flip-Flop1 : simulink_extras/Flip Flops/S-R Flip-Flop  initial_condition=0
  S-R Flip-Flop2 : simulink_extras/Flip Flops/S-R Flip-Flop  initial_condition=0
  Terminator : Terminator
  Terminator1 : Terminator
  Terminator2 : Terminator
  Out1 : Outport
  wires:
  Data Type Conversion/1 -> Out1/1
  Relational Operator/1 -> S-R Flip-Flop/1
  Constant1/1 -> S-R Flip-Flop/2, S-R Flip-Flop1/2, S-R Flip-Flop2/2
  RMS/1 -> Relational Operator/1
  S-R Flip-Flop1/2 -> Terminator1/1
  S-R Flip-Flop/2 -> Terminator/1
  S-R Flip-Flop2/2 -> Terminator2/1
  Iabc1/1 -> Demux/1
  Logical Operator/1 -> Data Type Conversion/1
  Constant/1 -> Relational Operator/2, Relational Operator1/2, Relational Operator2/2
  S-R Flip-Flop2/1 -> Logical Operator/3
  Relational Operator1/1 -> S-R Flip-Flop1/1
  S-R Flip-Flop/1 -> Logical Operator/1
  S-R Flip-Flop1/1 -> Logical Operator/2
  Relational Operator2/1 -> S-R Flip-Flop2/1
  Demux/1 -> RMS/1
  RMS2/1 -> Relational Operator1/1
  Demux/2 -> RMS2/1
  RMS1/1 -> Relational Operator2/1
  Demux/3 -> RMS1/1

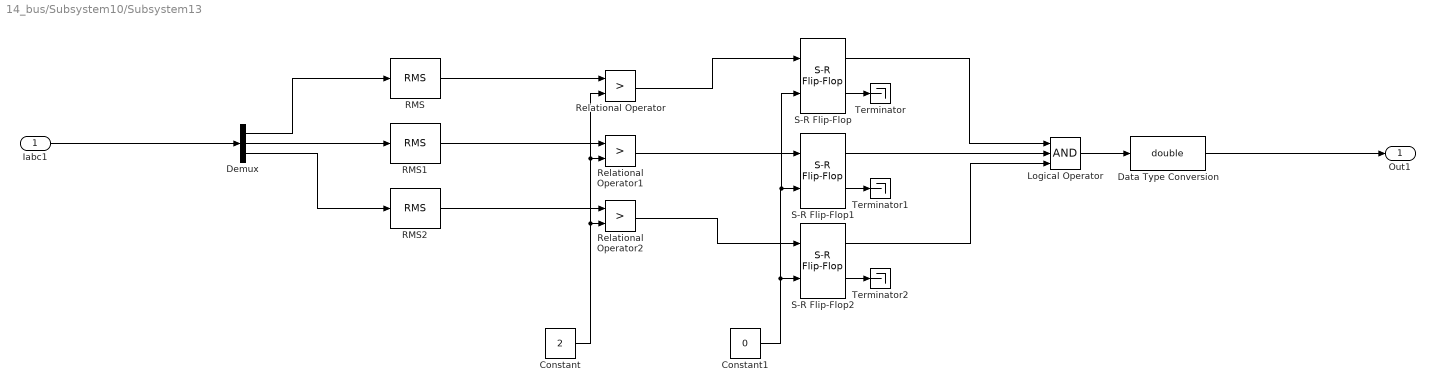
== system 14_bus/Subsystem10/Subsystem13 ==
  Iabc1 : Inport
  Constant : Constant  Value=2  OutDataTypeStr=boolean
  Constant1 : Constant  Value=0  OutDataTypeStr=boolean
  Data Type Conversion : DataTypeConversion  OutDataTypeStr=double  SaturateOnIntegerOverflow=off  RndMeth=Floor
  Demux : Demux  Outputs=3
  Logical Operator : Logic  Inputs=3  AllPortsSameDT=off  OutDataTypeStr=boolean
  RMS : spsRMSLib/RMS  TrueRMS=on  Freq=60  RMSInit=120  Ts=0
  RMS1 : spsRMSLib/RMS  TrueRMS=on  Freq=60  RMSInit=120  Ts=0
  RMS2 : spsRMSLib/RMS  TrueRMS=on  Freq=60  RMSInit=120  Ts=0
  Relational Operator : RelationalOperator  Operator=>  OutDataTypeStr=boolean  RndMeth=Simplest  InputSameDT=off
  Relational Operator1 : RelationalOperator  Operator=>  OutDataTypeStr=boolean  RndMeth=Simplest  InputSameDT=off
  Relational Operator2 : RelationalOperator  Operator=>  OutDataTypeStr=boolean  RndMeth=Simplest  InputSameDT=off
  S-R Flip-Flop : simulink_extras/Flip Flops/S-R Flip-Flop  initial_condition=0
  S-R Flip-Flop1 : simulink_extras/Flip Flops/S-R Flip-Flop  initial_condition=0
  S-R Flip-Flop2 : simulink_extras/Flip Flops/S-R Flip-Flop  initial_condition=0
  Terminator : Terminator
  Terminator1 : Terminator
  Terminator2 : Terminator
  Out1 : Outport
  wires:
  Data Type Conversion/1 -> Out1/1
  Relational Operator/1 -> S-R Flip-Flop/1
  Constant1/1 -> S-R Flip-Flop/2, S-R Flip-Flop1/2, S-R Flip-Flop2/2
  RMS/1 -> Relational Operator/1
  S-R Flip-Flop1/2 -> Terminator1/1
  S-R Flip-Flop/2 -> Terminator/1
  S-R Flip-Flop2/2 -> Terminator2/1
  Iabc1/1 -> Demux/1
  Logical Operator/1 -> Data Type Conversion/1
  Constant/1 -> Relational Operator/2, Relational Operator1/2, Relational Operator2/2
  S-R Flip-Flop2/1 -> Logical Operator/3
  Relational Operator1/1 -> S-R Flip-Flop1/1
  S-R Flip-Flop/1 -> Logical Operator/1
  S-R Flip-Flop1/1 -> Logical Operator/2
  Relational Operator2/1 -> S-R Flip-Flop2/1
  Demux/1 -> RMS/1
  RMS1/1 -> Relational Operator1/1
  Demux/2 -> RMS1/1
  RMS2/1 -> Relational Operator2/1
  Demux/3 -> RMS2/1

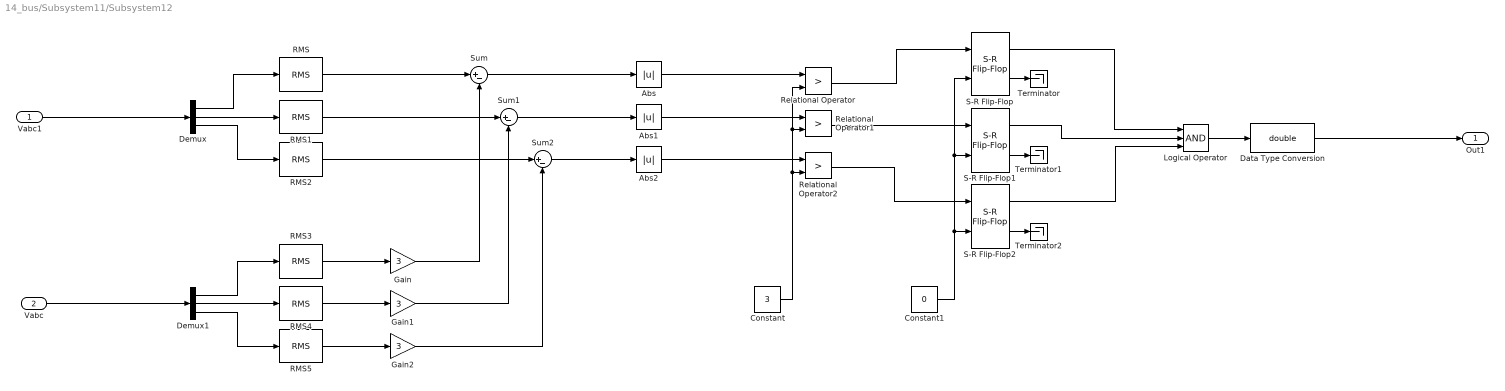
== system 14_bus/Subsystem11/Subsystem12 ==
  Vabc1 : Inport
  Vabc : Inport  Port=2
  Abs : Abs  SaturateOnIntegerOverflow=off
  Abs1 : Abs  SaturateOnIntegerOverflow=off
  Abs2 : Abs  SaturateOnIntegerOverflow=off
  Constant : Constant  Value=3  OutDataTypeStr=boolean
  Constant1 : Constant  Value=0  OutDataTypeStr=boolean
  Data Type Conversion : DataTypeConversion  OutDataTypeStr=double  SaturateOnIntegerOverflow=off  RndMeth=Floor
  Demux : Demux  Outputs=3
  Demux1 : Demux  Outputs=3
  Gain : Gain  Gain=3
  Gain1 : Gain  Gain=3
  Gain2 : Gain  Gain=3
  Logical Operator : Logic  Inputs=3  AllPortsSameDT=off  OutDataTypeStr=boolean
  RMS{,1..5} (6 alike) : spsRMSLib/RMS  TrueRMS=on  Freq=60  RMSInit=120  Ts=0
  Relational Operator : RelationalOperator  Operator=>  OutDataTypeStr=boolean  RndMeth=Simplest  InputSameDT=off
  Relational Operator1 : RelationalOperator  Operator=>  OutDataTypeStr=boolean  RndMeth=Simplest  InputSameDT=off
  Relational Operator2 : RelationalOperator  Operator=>  OutDataTypeStr=boolean  RndMeth=Simplest  InputSameDT=off
  S-R Flip-Flop : simulink_extras/Flip Flops/S-R Flip-Flop  initial_condition=0
  S-R Flip-Flop1 : simulink_extras/Flip Flops/S-R Flip-Flop  initial_condition=0
  S-R Flip-Flop2 : simulink_extras/Flip Flops/S-R Flip-Flop  initial_condition=0
  Sum : Sum  Inputs=|+-
  Sum1 : Sum  Inputs=|+-
  Sum2 : Sum  Inputs=|+-
  Terminator : Terminator
  Terminator1 : Terminator
  Terminator2 : Terminator
  Out1 : Outport
  wires:
  Sum1/1 -> Abs1/1
  RMS4/1 -> Gain1/1
  Sum/1 -> Abs/1
  RMS2/1 -> Sum2/1
  Abs/1 -> Relational Operator/1
  Relational Operator/1 -> S-R Flip-Flop/1
  Constant/1 -> Relational Operator/2, Relational Operator1/2, Relational Operator2/2
  RMS5/1 -> Gain2/1
  S-R Flip-Flop1/2 -> Terminator1/1
  Vabc1/1 -> Demux/1
  Demux1/3 -> RMS5/1
  RMS1/1 -> Sum1/1
  RMS/1 -> Sum/1
  RMS3/1 -> Gain/1
  Gain2/1 -> Sum2/2
  S-R Flip-Flop2/2 -> Terminator2/1
  Gain/1 -> Sum/2
  Abs2/1 -> Relational Operator2/1
  Demux/3 -> RMS2/1
  Demux1/2 -> RMS4/1
  Data Type Conversion/1 -> Out1/1
  Sum2/1 -> Abs2/1
  Constant1/1 -> S-R Flip-Flop/2, S-R Flip-Flop1/2, S-R Flip-Flop2/2
  Gain1/1 -> Sum1/2
  S-R Flip-Flop/1 -> Logical Operator/1
  Demux/1 -> RMS/1
  Demux1/1 -> RMS3/1
  Demux/2 -> RMS1/1
  S-R Flip-Flop1/1 -> Logical Operator/2
  Relational Operator2/1 -> S-R Flip-Flop2/1
  S-R Flip-Flop/2 -> Terminator/1
  Logical Operator/1 -> Data Type Conversion/1
  S-R Flip-Flop2/1 -> Logical Operator/3
  Relational Operator1/1 -> S-R Flip-Flop1/1
  Abs1/1 -> Relational Operator1/1
  Vabc/1 -> Demux1/1

== system 14_bus/Subsystem12/Subsystem1 ==
  Iabc1 : Inport
  Constant : Constant  Value=2  OutDataTypeStr=boolean
  Constant1 : Constant  Value=0  OutDataTypeStr=boolean
  Data Type Conversion : DataTypeConversion  OutDataTypeStr=double  SaturateOnIntegerOverflow=off  RndMeth=Floor
  Demux : Demux  Outputs=3
  Logical Operator : Logic  Inputs=3  AllPortsSameDT=off  OutDataTypeStr=boolean
  RMS : spsRMSLib/RMS  TrueRMS=on  Freq=60  RMSInit=120  Ts=0
  RMS1 : spsRMSLib/RMS  TrueRMS=on  Freq=60  RMSInit=120  Ts=0
  RMS2 : spsRMSLib/RMS  TrueRMS=on  Freq=60  RMSInit=120  Ts=0
  Relational Operator : RelationalOperator  Operator=>  OutDataTypeStr=boolean  RndMeth=Simplest  InputSameDT=off
  Relational Operator1 : RelationalOperator  Operator=>  OutDataTypeStr=boolean  RndMeth=Simplest  InputSameDT=off
  Relational Operator2 : RelationalOperator  Operator=>  OutDataTypeStr=boolean  RndMeth=Simplest  InputSameDT=off
  S-R Flip-Flop : simulink_extras/Flip Flops/S-R Flip-Flop  initial_condition=0
  S-R Flip-Flop1 : simulink_extras/Flip Flops/S-R Flip-Flop  initial_condition=0
  S-R Flip-Flop2 : simulink_extras/Flip Flops/S-R Flip-Flop  initial_condition=0
  Terminator : Terminator
  Terminator1 : Terminator
  Terminator2 : Terminator
  Out1 : Outport
  wires:
  Data Type Conversion/1 -> Out1/1
  Relational Operator/1 -> S-R Flip-Flop/1
  Constant1/1 -> S-R Flip-Flop/2, S-R Flip-Flop1/2, S-R Flip-Flop2/2
  RMS/1 -> Relational Operator/1
  S-R Flip-Flop1/2 -> Terminator1/1
  S-R Flip-Flop/2 -> Terminator/1
  S-R Flip-Flop2/2 -> Terminator2/1
  Iabc1/1 -> Demux/1
  Logical Operator/1 -> Data Type Conversion/1
  Constant/1 -> Relational Operator/2, Relational Operator1/2, Relational Operator2/2
  S-R Flip-Flop2/1 -> Logical Operator/3
  Relational Operator1/1 -> S-R Flip-Flop1/1
  S-R Flip-Flop/1 -> Logical Operator/1
  S-R Flip-Flop1/1 -> Logical Operator/2
  Relational Operator2/1 -> S-R Flip-Flop2/1
  Demux/1 -> RMS/1
  RMS1/1 -> Relational Operator1/1
  Demux/2 -> RMS1/1
  RMS2/1 -> Relational Operator2/1
  Demux/3 -> RMS2/1

== system 14_bus/Subsystem13/Subsystem1 ==
  Iabc1 : Inport
  Constant : Constant  Value=2  OutDataTypeStr=boolean
  Constant1 : Constant  Value=0  OutDataTypeStr=boolean
  Data Type Conversion : DataTypeConversion  OutDataTypeStr=double  SaturateOnIntegerOverflow=off  RndMeth=Floor
  Demux : Demux  Outputs=3
  Logical Operator : Logic  Inputs=3  AllPortsSameDT=off  OutDataTypeStr=boolean
  RMS : spsRMSLib/RMS  TrueRMS=on  Freq=60  RMSInit=120  Ts=0
  RMS1 : spsRMSLib/RMS  TrueRMS=on  Freq=60  RMSInit=120  Ts=0
  RMS2 : spsRMSLib/RMS  TrueRMS=on  Freq=60  RMSInit=120  Ts=0
  Relational Operator : RelationalOperator  Operator=>  OutDataTypeStr=boolean  RndMeth=Simplest  InputSameDT=off
  Relational Operator1 : RelationalOperator  Operator=>  OutDataTypeStr=boolean  RndMeth=Simplest  InputSameDT=off
  Relational Operator2 : RelationalOperator  Operator=>  OutDataTypeStr=boolean  RndMeth=Simplest  InputSameDT=off
  S-R Flip-Flop : simulink_extras/Flip Flops/S-R Flip-Flop  initial_condition=0
  S-R Flip-Flop1 : simulink_extras/Flip Flops/S-R Flip-Flop  initial_condition=0
  S-R Flip-Flop2 : simulink_extras/Flip Flops/S-R Flip-Flop  initial_condition=0
  Terminator : Terminator
  Terminator1 : Terminator
  Terminator2 : Terminator
  Out1 : Outport
  wires:
  Data Type Conversion/1 -> Out1/1
  Relational Operator/1 -> S-R Flip-Flop/1
  Constant1/1 -> S-R Flip-Flop/2, S-R Flip-Flop1/2, S-R Flip-Flop2/2
  RMS/1 -> Relational Operator/1
  S-R Flip-Flop1/2 -> Terminator1/1
  S-R Flip-Flop/2 -> Terminator/1
  S-R Flip-Flop2/2 -> Terminator2/1
  Iabc1/1 -> Demux/1
  Logical Operator/1 -> Data Type Conversion/1
  Constant/1 -> Relational Operator/2, Relational Operator1/2, Relational Operator2/2
  S-R Flip-Flop2/1 -> Logical Operator/3
  Relational Operator1/1 -> S-R Flip-Flop1/1
  S-R Flip-Flop/1 -> Logical Operator/1
  S-R Flip-Flop1/1 -> Logical Operator/2
  Relational Operator2/1 -> S-R Flip-Flop2/1
  Demux/1 -> RMS/1
  RMS1/1 -> Relational Operator1/1
  Demux/2 -> RMS1/1
  RMS2/1 -> Relational Operator2/1
  Demux/3 -> RMS2/1
